simulink library "INT_FlSys_FlCons"  (R2016b)
settings: Solver=VariableStepAuto  StartTime=0.0  StopTime=10.0  RelTol=1e-3
settings Model: Creator=Administrator  LastModifiedBy=Administrator

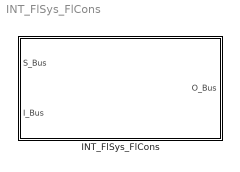
== system INT_FlSys_FlCons ==
  INT_FlSys_FlCons : Subsystem

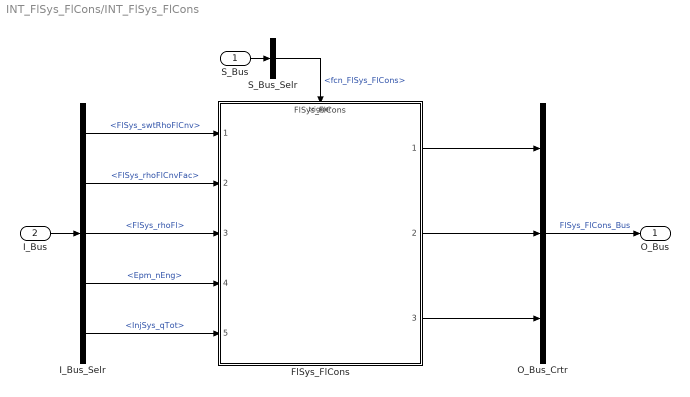
== system INT_FlSys_FlCons/INT_FlSys_FlCons ==
  S_Bus : Inport
  I_Bus : Inport  Port=2
  FlSys_FlCons : ModelReference  ModelNameDialog=FlSys_FlCons  SimulationMode=Normal  ModelReferenceVersion=1.6  TriggerPortName=function  TriggerPortTriggerType=function-call  TriggerPortStatesWhenEnabling=held
  I_Bus_Selr : BusSelector  OutputSignals=FlSys_swtRhoFlCnv,FlSys_rhoFlCnvFac,FlSys_rhoFl,Epm_nEng,InjSys_qTot
  O_Bus_Crtr : BusCreator  Inputs=3
  S_Bus_Selr : BusSelector  OutputSignals=fcn_FlSys_FlCons
  O_Bus : Outport
  wires:
  S_Bus_Selr/1 -> FlSys_FlCons/Trigger  "<fcn_FlSys_FlCons>"
  S_Bus/1 -> S_Bus_Selr/1
  I_Bus/1 -> I_Bus_Selr/1
  I_Bus_Selr/1 -> FlSys_FlCons/1  "<FlSys_swtRhoFlCnv>"
  I_Bus_Selr/2 -> FlSys_FlCons/2  "<FlSys_rhoFlCnvFac>"
  I_Bus_Selr/3 -> FlSys_FlCons/3  "<FlSys_rhoFl>"
  I_Bus_Selr/4 -> FlSys_FlCons/4  "<Epm_nEng>"
  I_Bus_Selr/5 -> FlSys_FlCons/5  "<InjSys_qTot>"
  O_Bus_Crtr/1 -> O_Bus/1  "FlSys_FlCons_Bus"
  FlSys_FlCons/1 -> O_Bus_Crtr/1
  FlSys_FlCons/2 -> O_Bus_Crtr/2
  FlSys_FlCons/3 -> O_Bus_Crtr/3
